simulink model "Test1"  (R2020b)
settings: Solver=ode3  StartTime=0.0  StopTime=10  RelTol=1e-3  EnableMultiTasking=on
libraries: arduinolib x4, simulink x1, arduinosensorlib x1
settings Model: FPTRunName=Active  SILPILModeSetting=veronly  ExtModeTrigDuration=2  Creator=ignaI  LastModifiedBy=ignaI
settings DataIOCC: LimitDataPoints=on  SaveFormat=Array
settings OptimizationCC: ExpressionDepthLimit=2147483647  LifeSpan=Inf  MaxStackSize=64
settings DebuggingCC: UnderspecifiedInitializationDetection=Classic  MergeDetectMultiDrivingBlocksExec=none  FcnCallInpInsideContextMsg=warning  AllowSymbolicDim=off  StateNameClashWarn=warning  SFUnexpectedBacktrackingDiag=warning  SFNoUnconditionalDefaultTransitionDiag=warning  SFExecutionAtInitializationDiag=none  ArithmeticOperatorsInVariantConditions=warning
settings HardwareCC: ProdBitPerInt=16  ProdBitPerPointer=16  ProdBitPerSizeT=16  ProdBitPerPtrDiffT=16  ProdLargestAtomicFloat=None  ProdWordSize=8  ProdHWDeviceType=Atmel->AVR  UseEmbeddedCoderFeatures=off  UseSimulinkCoderFeatures=off
settings ModelReferenceCC: PropagateSignalLabelsOutOfModel=off
settings SFSimCC: SimUseLocalCustomCode=off  CustomCodeUndefinedFunction=UseInterfaceOnly
settings RTWCC: Description=Embedded Coder  SystemTargetFile=ert.tlc  HardwareBoard=Arduino Uno  TemplateMakefile=ert_default_tmf  GenerateReport=on  RTWVerbose=off  RTWUseLocalCustomCode=off  Toolchain=Arduino AVR  BuildConfiguration=Faster Runs  LaunchReport=on
settings CodeAppCC: ForceParamTrailComments=on  OperatorAnnotations=on  MangleLength=10  StateflowObjectComments=on  MATLABSourceComments=on
settings ERTTargetCC: MultiwordLength=2048  ERTCustomFileBanners=off  SupportContinuousTime=on  SupportNonInlinedSFcns=on  RemoveResetFunc=off  SupportVariableSizeSignals=on  ModelStepFunctionPrototypeControlCompliant=off  ExtModeStaticAllocSize=250
settings ConfigComp: CovMetricSettings=dw  CovSaveCumulativeToWorkspaceVar=on  CovSaveSingleToWorkspaceVar=on  CovExternalEMLEnable=off  CovSFcnEnable=off

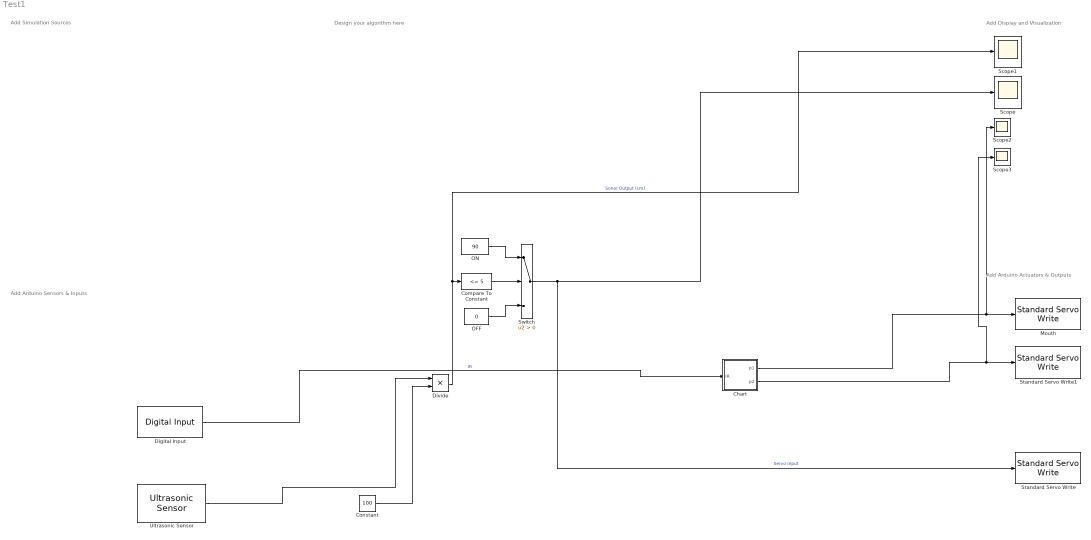
== system Test1 ==
  note: Add Arduino Actuators & Outputs
  note: Add Arduino Sensors & Inputs
  note: Design your algorithm here
  note: Add Display and Visualization
  note: Add Simulation Sources
  Chart : Stateflow chart  TreatAsAtomicUnit=on
  Compare To Constant : simulink/Logic and Bit Operations/Compare To Constant  relop=<=  const=5  OutDataTypeStr=boolean
  Constant : Constant  Value=100  SampleTime=-1
  Digital Input : arduinolib/Digital Input  pinNumber=8  mode=Default  Direction=input  SampleTime=0.1  blockPlatform=arduino
  Divide : Product  Inputs=**
  Mouth : arduinolib/Standard Servo Write  pinNumber=7  ServoIndex=0  blockPlatform=ARDUINO
  OFF : Constant  Value=0  SampleTime=-1
  ON : Constant  Value=90  SampleTime=-1
  Scope{,1..3} (4 alike) : Scope
  Standard Servo Write : arduinolib/Standard Servo Write  pinNumber=9  ServoIndex=1  blockPlatform=ARDUINO
  Standard Servo Write1 : arduinolib/Standard Servo Write  pinNumber=6  ServoIndex=2  blockPlatform=ARDUINO
  Switch : Switch  Criteria=u2 > Threshold
  Ultrasonic Sensor : arduinosensorlib/Ultrasonic Sensor  NumSignalPins=2  TrigPin=4  EchoPin=5  SignalPin=3  SampleTime_=0.1  blockPlatform=ARDUINO
      settings: SourceProductBaseCode=ARDUINO
  wires:
  ON/1 -> Switch/1
  Compare To Constant/1 -> Switch/2
  OFF/1 -> Switch/3
  Switch/1 -> Standard Servo Write/1, Scope/1  "Servo Input"
  Constant/1 -> Divide/2
  Ultrasonic Sensor/1 -> Divide/1
  Divide/1 -> Compare To Constant/1, Scope1/1  "Sonar Output (cm)"
  Digital Input/1 -> Chart/1(IR)  "IR"
  Chart/1(p1) -> Scope2/1, Mouth/1
  Chart/2(p2) -> Scope3/1, Standard Servo Write1/1

== stateflow chart Test1/Chart ==
  state INIT
  state N1
  state N2
  (default) -> INIT
  INIT -> N1 : {p1=0,p2=0}
  N1 -> N2 : [IR]{p1=90,p2=45}
  N2 -> N1 : [~IR]{p1=45,p2=90}
  data: IR input; p1 output; p2 output
